simulink model "zad3"  (R2017a)
settings: Solver=VariableStepAuto  StartTime=0.0  StopTime=10.0  RelTol=1e-3
settings Model: Creator=DoktorHax  LastModifiedBy=DoktorHax

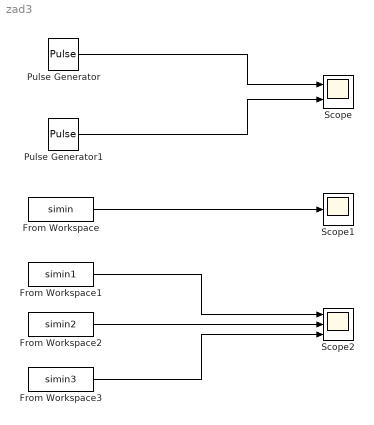
== system zad3 ==
  From Workspace : FromWorkspace  VariableName=simin  SampleTime=0  Interpolate=off  OutputAfterFinalValue=Holding final value
  From Workspace1 : FromWorkspace  VariableName=simin1  SampleTime=0  Interpolate=off  OutputAfterFinalValue=Holding final value
  From Workspace2 : FromWorkspace  VariableName=simin2  SampleTime=0  Interpolate=off  OutputAfterFinalValue=Holding final value
  From Workspace3 : FromWorkspace  VariableName=simin3  SampleTime=0  Interpolate=off  OutputAfterFinalValue=Holding final value
  Pulse Generator : DiscretePulseGenerator  PulseType=Time based  PulseWidth=50  PhaseDelay=1
  Pulse Generator1 : DiscretePulseGenerator  PulseType=Time based  Period=4  PulseWidth=50  PhaseDelay=2
  Scope : Scope  NumInputPorts=2
  Scope1 : Scope
  Scope2 : Scope  NumInputPorts=3
  wires:
  Pulse Generator/1 -> Scope/1
  Pulse Generator1/1 -> Scope/2
  From Workspace/1 -> Scope1/1
  From Workspace1/1 -> Scope2/1
  From Workspace2/1 -> Scope2/2
  From Workspace3/1 -> Scope2/3
